simulink model "SecOrdMdl_Prototype"  (R2023b)
settings: Solver=ode8  StartTime=0.0  StopTime=5  FixedStep=1e-3  RelTol=1e-3
values from neighbouring files (symbols this model uses):
  J = Jr/(Ng^2) + Jg    [SecondOrderModel.m]
  K = lqr(A,B,Q,R)    [SecondOrderModel.m]
  Tg = Dg*s    [SecondOrderModel.m]
  u0 = 11.9    [SecondOrderModel.m]
  x0 = [omega_g0; u0]    [SecondOrderModel.m]
undefined symbols (not defined in the file or in its folder): Dg, Ng, omega_0, p, tau_theta, theta_dot_max, theta_max, theta_min
libraries: slpidlib x1, simulink x1
settings Model: Creator=Selim  LastModifiedBy=Selim

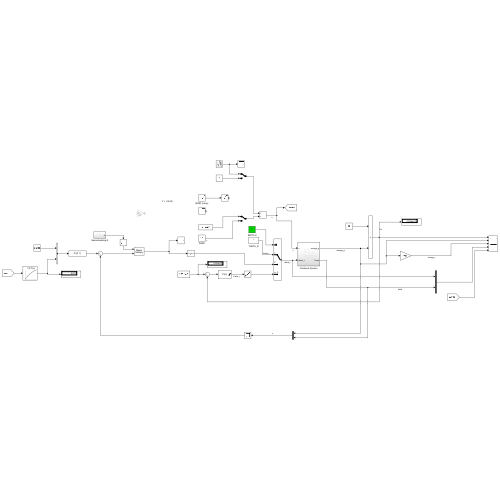
[thumbnail: Simulink's stored preview of the top-level diagram]
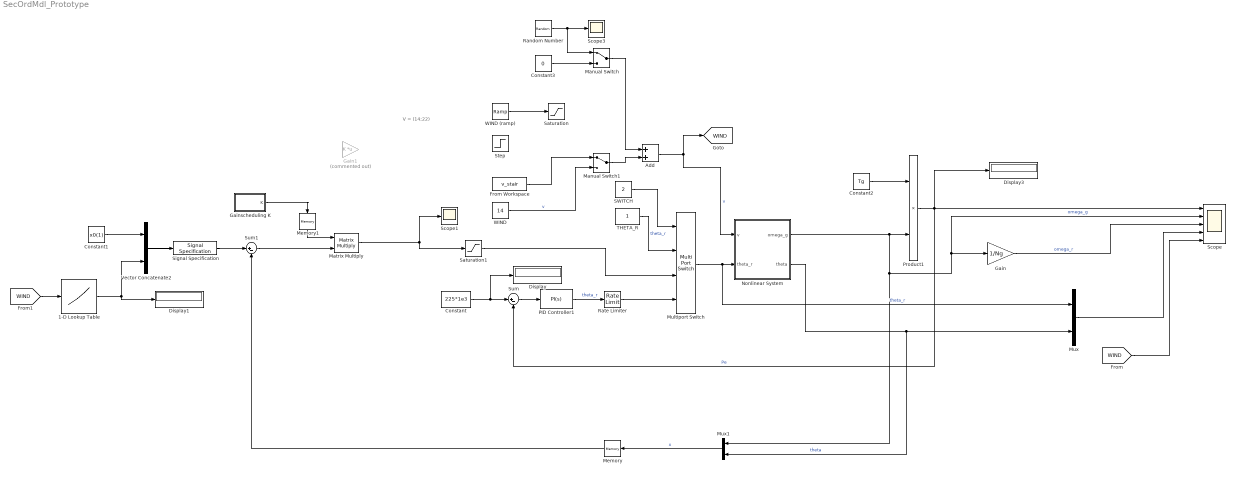
== system SecOrdMdl_Prototype ==
  note: V = (14;22)
  1-D Lookup Table : Lookup_n-D  NumberOfTableDimensions=1  BreakpointsForDimension1=[14 16 18 20 22]  Table=[11.9 16.2 19.1 21.2 22.8]  InternalRulePriority=Speed  RndMeth=Simplest
  Add : Sum
  Constant : Constant  Value=225*1e3
  Constant1 : Constant  Value=x0(1)
  Constant2 : Constant  Value=Tg
  Constant3 : Constant  Value=0
  Display : Display
  Display1 : Display
  Display3 : Display
  From Workspace : FromWorkspace  VariableName=v_stair
  Gain : Gain  Gain=1/Ng
  Gain1 : Gain  Commented=on  Gain=K  Multiplication=Matrix(K*u)
  Gainscheduling K : Subsystem
  Manual Switch : ManualSwitch
  Manual Switch1 : ManualSwitch
  Matrix Multiply : Product  Multiplication=Matrix(*)
  Memory : Memory  InitialCondition=x0
  Memory1 : Memory  InitialCondition=K
  Multiport Switch : MultiPortSwitch  SaturateOnIntegerOverflow=off  InputSameDT=off
  Mux : Mux  Inputs=2
  Mux1 : Mux  Inputs=2
  Nonlinear System : Subsystem
  PID Controller1 : slpidlib/PID Controller  Controller=PI  Form=Parallel  TimeDomain=Continuous-time  UseExternalTs=off  SampleTime=-1  IntegratorMethod=Forward Euler  FilterMethod=Forward Euler  ControllerParametersSource=internal  P=-6.03660291875363e-05  I=-0.00249732862255308  UseKiTs=off  D=-0.00034354310668366  N=1044.45037459015  UseFilter=on  TunerSelectOption=Transfer Function Based (PID Tuner App)  InitialConditionSource=internal  InitialConditionForIntegrator=0  InitialConditionForFilter=0  DifferentiatorICPrevScaledInput=0  ExternalReset=none  TrackingMode=off  Kt=1  LimitOutput=on  SatLimitsSource=internal  UpperSaturationLimit=theta_max  LowerSaturationLimit=theta_min  LinearizeAsGain=on  AntiWindupMode=clamping  Kb=1  LimitIntegrator=off  UpperIntegratorSaturationLimit=inf  LowerIntegratorSaturationLimit=-inf  POutMin=[]  POutMax=[]  IOutMin=[]  IOutMax=[]  DOutMin=[]  DOutMax=[]  NOutMin=[]  NOutMax=[]  SumOutMin=[]  SumOutMax=[]  SaturationOutMin=[]  SaturationOutMax=[]  PParamMin=[]  PParamMax=[]  IParamMin=[]  IParamMax=[]  DParamMin=[]  DParamMax=[]  NParamMin=[]  NParamMax=[]  KbParamMin=[]  KbParamMax=[]  KtParamMin=[]  KtParamMax=[]  KbOutMin=[]  KbOutMax=[]  KtOutMin=[]  KtOutMax=[]  IntegratorOutMin=[]  IntegratorOutMax=[]  FilterOutMin=[]  FilterOutMax=[]  SumI1OutMin=[]  SumI1OutMax=[]  SumI2OutMin=[]  SumI2OutMax=[]  SumI3OutMin=[]  SumI3OutMax=[]  SumI4OutMin=[]  SumI4OutMax=[]  SumDOutMin=[]  SumDOutMax=[]  DifferentiatorOutMin=[]  DifferentiatorOutMax=[]  FilterDiffOutCoefMin=[]  FilterDiffOutCoefMax=[]  ReciprocalOutMin=[]  ReciprocalOutMax=[]  SumDenOutMin=[]  SumDenOutMax=[]  SumNumOutMin=[]  SumNumOutMax=[]  DivideOutMin=[]  DivideOutMax=[]  UdiffTsProdOutMin=[]  UdiffTsProdOutMax=[]  NTsProdOutMin=[]  NTsProdOutMax=[]  UintegralTsProdOutMin=[]  UintegralTsProdOutMax=[]  UngainTsProdOutMin=[]  UngainTsProdOutMax=[]  ClampingZeroOutDataTypeStr=Inherit: Inherit via back propagation  ClampingZeroOutMin=[]  ClampingZeroOutMax=[]  FilterDenConstantOutDataTypeStr=Inherit: Inherit via back propagation  FilterDenConstantOutMin=[]  FilterDenConstantOutMax=[]  PCopyOutDataTypeStr=Inherit: Inherit via back propagation  PCopyOutMin=[]  PCopyOutMax=[]  NCopyOutDataTypeStr=Inherit: Inherit via back propagation  NCopyOutMin=[]  NCopyOutMax=[]  IntegratorContinuousStateAttributes=''  IntegratorStateMustResolveToSignalObject=off  IntegratorRTWStateStorageClass=Auto  FilterContinuousStateAttributes=''  FilterStateMustResolveToSignalObject=off  FilterRTWStateStorageClass=Auto  ParallelPVariant=InternalParameters  IdealPVariant=Disabled  IVariant=InternalParameters  DVariant=Disabled  IntegratorVariant=Continuous  SatVariant=Enabled  AWVariant=ContClampingParallel  PCopyVariant=Disabled  TRVariant=Disabled  FdbkBlocksVariant=Forward  IdealPFdbkVariant=Disabled  SatFdbkVariant=Disabled  DerivativeFilterVariant=Disabled  NVariant=Disabled  NCopyVariant=Disabled_SignalSpec  FilterICVariant=Disabled  IntegratorICVariant=InternalICs  ExternalResetVariant=Disabled  TRSumVariant=Passthrough  SumFdbkVariant=Disabled  SumVariant=Sum_PI  TsampFilterVariant=InternalTs  TsampNgainVariant=Passthrough  TsampIntegralVariant=Disabled_SignalSpec  ExternalSaturationOutDataTypeStr=Inherit: Same as second input
  Product1 : Product
  Random Number : RandomNumber  SampleTime=1e-2
  Rate Limiter : RateLimiter  RisingSlewLimit=theta_dot_max  FallingSlewLimit=-theta_dot_max  SampleTimeMode=inherited
  SWITCH : Constant  Value=2
  Saturation : Saturate  UpperLimit=22  LowerLimit=12
  Saturation1 : Saturate  UpperLimit=theta_max  LowerLimit=theta_min
  Scope : Scope  NumInputPorts=5
  Scope1 : Scope
  Scope3 : Scope
  Signal Specification : SignalSpecification  Dimensions=[2 1]
  Step : Step  Before=14  After=22  SampleTime=0
  Sum : Sum  Inputs=|+-
  Sum1 : Sum  Inputs=|+-
  THETA_R : Constant
  Vector Concatenate2 : Concatenate
  WIND : Constant  Value=14
  WIND (ramp) : simulink/Sources/Ramp  slope=3  start=1  InitialOutput=14
  tag scope: WIND=global
  wires:
  Add/1 -> Nonlinear System/1(v), [WIND]  "v"
  PID Controller1/1 -> Rate Limiter/1  "theta_r"
  Nonlinear System/2(theta) -> Mux1/2, Mux/2  "theta"
  Nonlinear System/1(omega_g) -> Mux1/1, Scope/2, Gain/1, Product1/2  "omega_g"
  Product1/1 -> Display3/1, Scope/1, Sum/2  "Pe"
  Sum/1 -> PID Controller1/1
  Constant/1 -> Display/1, Sum/1
  THETA_R/1 -> Multiport Switch/2  "theta_r"
  Multiport Switch/1 -> Mux/1, Nonlinear System/2(theta_r)  "theta_r"
  Constant2/1 -> Product1/1
  Gain/1 -> Scope/3  "omega_r"
  Mux/1 -> Scope/4
  Rate Limiter/1 -> Multiport Switch/4
  Random Number/1 -> Manual Switch/1, Scope3/1
  SWITCH/1 -> Multiport Switch/1
  Mux1/1 -> Memory/1  "x"
  Vector Concatenate2/1 -> Signal Specification/1
  Sum1/1 -> Matrix Multiply/2
  Matrix Multiply/1 -> Saturation1/1, Scope1/1
  Manual Switch/1 -> Add/1
  Constant3/1 -> Manual Switch/2
  [WIND] -> Scope/5
  WIND/1 -> Manual Switch1/2  "v"
  WIND (ramp)/1 -> Saturation/1
  Manual Switch1/1 -> Add/2
  Memory/1 -> Sum1/2
  Saturation1/1 -> Multiport Switch/3
  Constant1/1 -> Vector Concatenate2/1
  [WIND] -> 1-D Lookup Table/1
  1-D Lookup Table/1 -> Display1/1, Vector Concatenate2/2
  Signal Specification/1 -> Sum1/1
  Gainscheduling K/1(K) -> Memory1/1
  Memory1/1 -> Matrix Multiply/1
  From Workspace/1 -> Manual Switch1/1

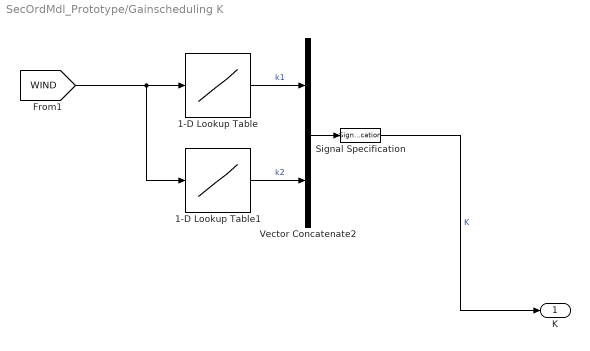
== system SecOrdMdl_Prototype/Gainscheduling K ==
  1-D Lookup Table : Lookup_n-D  NumberOfTableDimensions=1  BreakpointsForDimension1=[14 16 18 20 22]  Table=[0.1658 0.0683 0.0367 0.0229 0.0155]  InternalRulePriority=Speed  RndMeth=Simplest
  1-D Lookup Table1 : Lookup_n-D  NumberOfTableDimensions=1  BreakpointsForDimension1=[14 16 18 20 22]  Table=[8.1869 20.6413 35.2098 52.5979 73.7912]  InternalRulePriority=Speed  RndMeth=Simplest
  Signal Specification : SignalSpecification  Dimensions=[1 2]
  Vector Concatenate2 : Concatenate
  K : Outport
  wires:
  Vector Concatenate2/1 -> Signal Specification/1
  1-D Lookup Table/1 -> Vector Concatenate2/1  "k1"
  1-D Lookup Table1/1 -> Vector Concatenate2/2  "k2"
  [WIND] -> 1-D Lookup Table1/1, 1-D Lookup Table/1
  Signal Specification/1 -> K/1  "K"

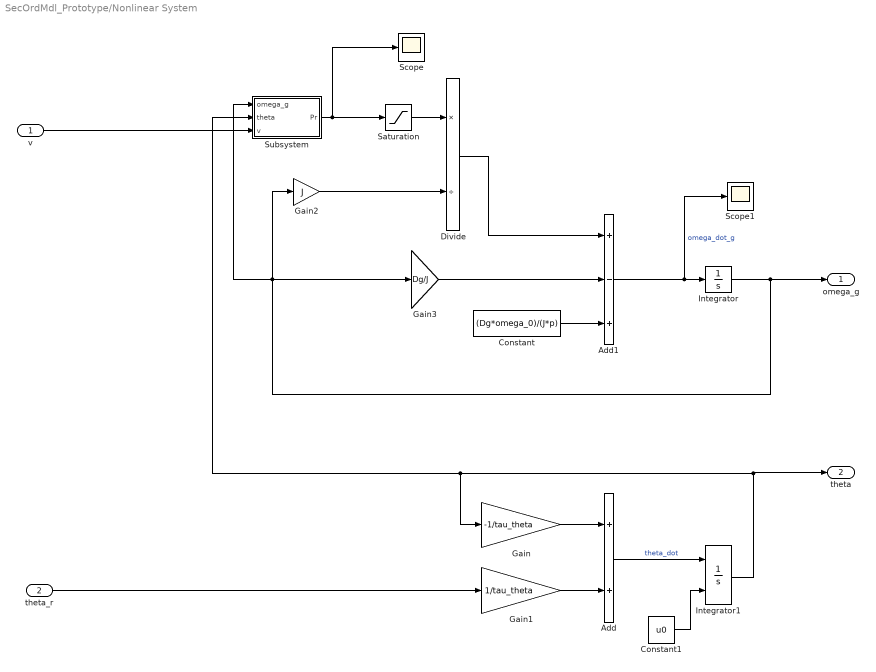
== system SecOrdMdl_Prototype/Nonlinear System ==
  v : Inport
  theta_r : Inport  Port=2
  Add : Sum
  Add1 : Sum  Inputs=+-+
  Constant : Constant  Value=(Dg*omega_0)/(J*p)
  Constant1 : Constant  Value=u0
  Divide : Product  Inputs=*/
  Gain : Gain  Gain=-1/tau_theta
  Gain1 : Gain  Gain=1/tau_theta
  Gain2 : Gain  Gain=J
  Gain3 : Gain  Gain=Dg/J
  Integrator : Integrator  InitialCondition=x0(1)
  Integrator1 : Integrator  InitialConditionSource=external  InitialCondition=1
  Saturation : Saturate  UpperLimit=inf  LowerLimit=1
  Scope : Scope
  Scope1 : Scope
  Subsystem : Subsystem
  omega_g : Outport
  theta : Outport  Port=2
  wires:
  Gain3/1 -> Add1/2
  Integrator/1 -> Subsystem/1(omega_g), Gain3/1, Gain2/1, omega_g/1
  Integrator1/1 -> Subsystem/2(theta), Gain/1, theta/1
  Constant/1 -> Add1/3
  Gain/1 -> Add/1
  Subsystem/1(Pr) -> Scope/1, Saturation/1
  Gain1/1 -> Add/2
  Gain2/1 -> Divide/2
  Divide/1 -> Add1/1
  v/1 -> Subsystem/3(v)
  Add1/1 -> Scope1/1, Integrator/1  "omega_dot_g"
  Add/1 -> Integrator1/1  "theta_dot"
  theta_r/1 -> Gain1/1
  Saturation/1 -> Divide/1
  Constant1/1 -> Integrator1/2

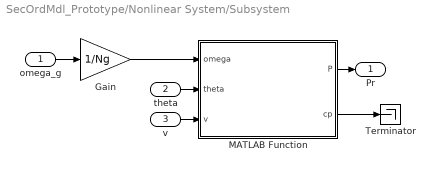
== system SecOrdMdl_Prototype/Nonlinear System/Subsystem ==
  omega_g : Inport
  theta : Inport  Port=2
  v : Inport  Port=3
  Gain : Gain  Gain=1/Ng
  MATLAB Function : MATLAB Function  TreatAsAtomicUnit=on
  Terminator : Terminator
  Pr : Outport
  wires:
  theta/1 -> MATLAB Function/2(theta)
  MATLAB Function/2(cp) -> Terminator/1
  MATLAB Function/1(P) -> Pr/1
  v/1 -> MATLAB Function/3(v)
  omega_g/1 -> Gain/1
  Gain/1 -> MATLAB Function/1(omega)

== matlab function SecOrdMdl_Prototype/Nonlinear System/Subsystem/MATLAB Function ==
  data: omega input; P output; theta input; v input; cp output
function [P,cp] = getAerodynamics(omega,theta,v)

R = 14.5;
rho = 1.2;

lambda = v/(R*omega);
lambda_t = 1/(1/(lambda^-1 + 0.12*theta) - 0.0035/((1.5*theta)^3 + 1));

cp = 0.22*(116/lambda_t - 0.6*theta - 5)*exp(-12.5/lambda_t);

P = 1/2*rho*pi*(R^2)*(v^3)*abs(cp);
